simulink model "sistema1"  (R2023a)
settings: Solver=ode23t  StartTime=0.0  StopTime=10.0  MaxStep=1E-3  RelTol=1e-3
libraries: simulink x1
settings Model: LastModifiedBy=anada
settings DataIOCC: ReturnWorkspaceOutputs=off  TimeSaveName=t
settings DebuggingCC: AlgebraicLoopMsg=none  ArtificialAlgebraicLoopMsg=none  MaxConsecutiveZCsMsg=none
settings RTWCC: GPUComputeCapability=5.0

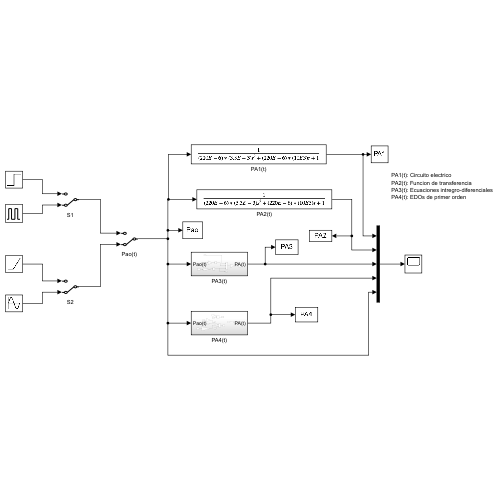
[thumbnail: Simulink's stored preview of the top-level diagram]
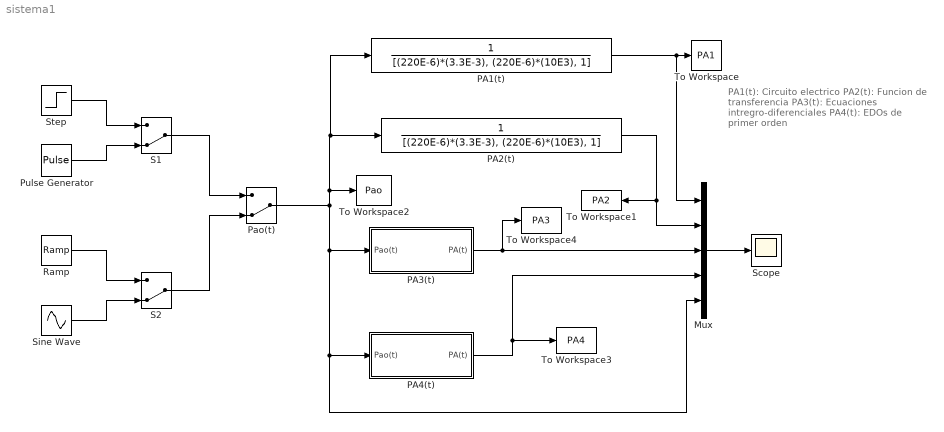
== system sistema1 ==
  note: PA1(t): Circuito electrico
      | PA2(t): Funcion de transferencia
      | PA3(t): Ecuaciones intregro-diferenciales
      | PA4(t): EDOs de primer orden
  Mux : Mux  Inputs=5
  PA1(t) : TransferFcn  Denominator=[(220E-6)*(3.3E-3), (220E-6)*(10E3), 1]
  PA2(t) : TransferFcn  Denominator=[(220E-6)*(3.3E-3), (220E-6)*(10E3), 1]
  PA3(t) : Subsystem
  PA4(t) : Subsystem
  Pao(t) : ManualSwitch  CurrentSetting=0
  Pulse Generator : DiscretePulseGenerator  PulseType=Time based  Period=10  PulseWidth=10  PhaseDelay=1
  Ramp : simulink/Sources/Ramp  slope=1/10  start=0  InitialOutput=0
  S1 : ManualSwitch  CurrentSetting=0
  S2 : ManualSwitch  CurrentSetting=0
  Scope : Scope
  Sine Wave : Sin  Frequency=pi/2  SampleTime=0
  Step : Step  Time=0  Before=1  SampleTime=0
  To Workspace : ToWorkspace  VariableName=PA1  SampleTime=-1
  To Workspace1 : ToWorkspace  VariableName=PA2  SampleTime=-1
  To Workspace2 : ToWorkspace  VariableName=Pao  SampleTime=-1
  To Workspace3 : ToWorkspace  VariableName=PA4  SampleTime=-1
  To Workspace4 : ToWorkspace  VariableName=PA3  SampleTime=-1
  wires:
  Step/1 -> S1/1
  S1/1 -> Pao(t)/1
  Pao(t)/1 -> PA3(t)/1(Pao(t)), PA4(t)/1(Pao(t)), Mux/5, To Workspace2/1, PA1(t)/1, PA2(t)/1
  S2/1 -> Pao(t)/2
  Pulse Generator/1 -> S1/2
  Ramp/1 -> S2/1
  Sine Wave/1 -> S2/2
  PA4(t)/1(PA(t)) -> To Workspace3/1, Mux/4
  PA3(t)/1(PA(t)) -> To Workspace4/1, Mux/3
  PA2(t)/1 -> To Workspace1/1, Mux/2
  Mux/1 -> Scope/1
  PA1(t)/1 -> Mux/1, To Workspace/1

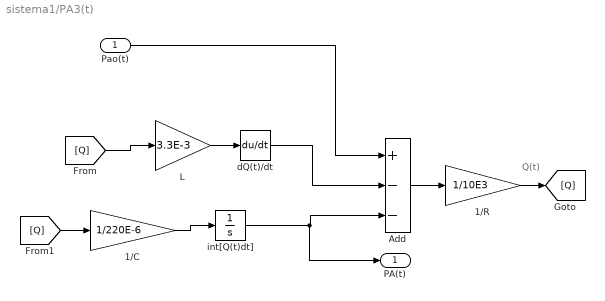
== system sistema1/PA3(t) ==
  note: Q(t)
  Pao(t) : Inport
  1/C : Gain  Gain=1/220E-6
  1/R : Gain  Gain=1/10E3
  Add : Sum  Inputs=+--
  L : Gain  Gain=3.3E-3
  dQ(t)/dt : Derivative
  int[Q(t)dt] : Integrator
  PA(t) : Outport
  wires:
  dQ(t)/dt/1 -> Add/2
  L/1 -> dQ(t)/dt/1
  Pao(t)/1 -> Add/1
  int[Q(t)dt]/1 -> PA(t)/1, Add/3
  1/C/1 -> int[Q(t)dt]/1
  [Q] -> L/1
  [Q] -> 1/C/1
  Add/1 -> 1/R/1
  1/R/1 -> [Q]

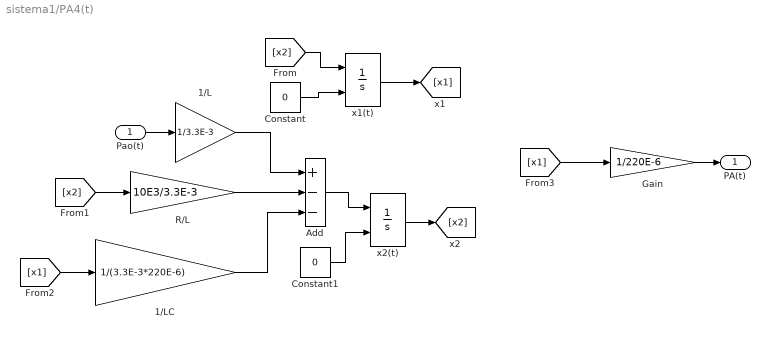
== system sistema1/PA4(t) ==
  Pao(t) : Inport
  1/L : Gain  Gain=1/3.3E-3
  1/LC : Gain  Gain=1/(3.3E-3*220E-6)
  Add : Sum  Inputs=+--
  Constant : Constant  Value=0
  Constant1 : Constant  Value=0
  Gain : Gain  Gain=1/220E-6
  R/L : Gain  Gain=10E3/3.3E-3
  x1(t) : Integrator  InitialConditionSource=external
  x2(t) : Integrator  InitialConditionSource=external
  PA(t) : Outport
  wires:
  [x2] -> x1(t)/1
  x1(t)/1 -> [x1]
  Constant/1 -> x1(t)/2
  x2(t)/1 -> [x2]
  Constant1/1 -> x2(t)/2
  Add/1 -> x2(t)/1
  Pao(t)/1 -> 1/L/1
  1/L/1 -> Add/1
  R/L/1 -> Add/2
  [x2] -> R/L/1
  1/LC/1 -> Add/3
  [x1] -> 1/LC/1
  [x1] -> Gain/1
  Gain/1 -> PA(t)/1
